simulink subsystem "Plant_PlantWithPressureBus"  (R2023a)
settings: Solver=VariableStepAuto  StartTime=0.0  StopTime=10.0  RelTol=1e-3
settings Model: Creator=giaco  LastModifiedBy=giaco

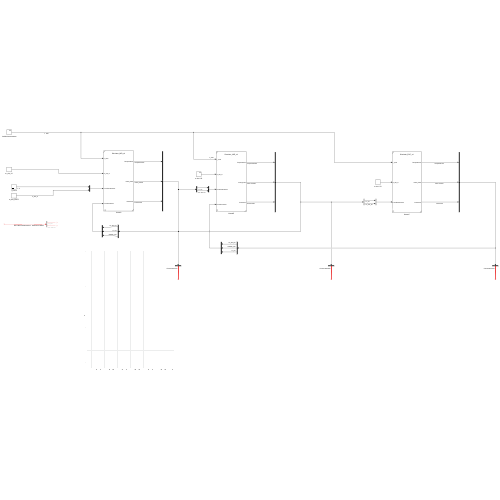
[thumbnail: Simulink's stored preview of the top-level diagram]
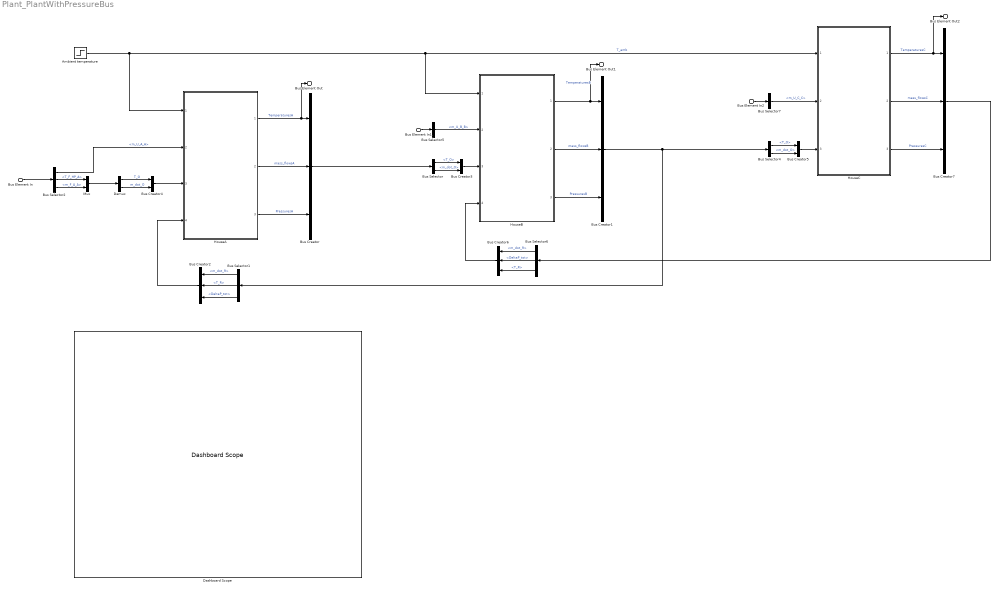
== system Plant_PlantWithPressureBus ==
  Bus Element In : Inport  PortName=InSim  Element=HouseA
  Bus Element In1 : Inport  PortName=InSim  Element=HouseB
  Bus Element In2 : Inport  PortName=InSim  Element=HouseC
  Ambient temperature : Step  Time=0  Before=300  After=300  SampleTime=0
  Bus Creator{,1..2,6..7} (5 alike) : BusCreator  Inputs=3
  Bus Creator3 : BusCreator  Inputs=2
  Bus Creator4 : BusCreator  Inputs=2
  Bus Creator5 : BusCreator  Inputs=2
  Bus Selector : BusSelector  OutputSignals=TemperaturesA.T_O,mass_flowsA.m_dot_O
  Bus Selector1 : BusSelector  OutputSignals=mass_flowsB.m_dot_R,TemperaturesB.T_R,PressuresB.DeltaP_tot
  Bus Selector2 : BusSelector  OutputSignals=m_U_A_A,T_F_HP_A,m_F_A_A
  Bus Selector4 : BusSelector  OutputSignals=TemperaturesB.T_O,mass_flowsB.m_dot_O
  Bus Selector5 : BusSelector  OutputSignals=m_U_B_B
  Bus Selector6 : BusSelector  OutputSignals=mass_flowsC.m_dot_R,PressuresC.DeltaP_tot,TemperaturesC.T_R
  Bus Selector7 : BusSelector  OutputSignals=m_U_C_C
  Dashboard Scope : DashboardScope
  Demux : Demux  Outputs=2
  HouseA : Subsystem  ReferencedSubsystem=Simulator_MID_v4  rho=971  c_p=4179  pi=3.14151  f_Darcy=0.025  L_F=40.5  D_F=0.4  h_F=1.5  D_S1=1  L_S1=0.4  h_S1=1.5  D_S2=0.4  L_S2=50  h_S2=1.5  D_S3=0.4  L_S3=5  h_S3=1.5  D_R=0.4  L_R=40  h_R=1.5  C_b=300  A_b=500  h_b=1.5  T_F_0=273  T_S1_0=273  T_S2_0=273  T_S3_0=273  T_b_0=273  T_R_0=273
  HouseB : Subsystem  ReferencedSubsystem=Simulator_MID_v4  rho=971  c_p=4179  pi=3.14151  f_Darcy=0.025  L_F=40.5  D_F=0.4  h_F=1.5  D_S1=1  L_S1=0.4  h_S1=1.5  D_S2=0.4  L_S2=50  h_S2=1.5  D_S3=0.4  L_S3=5  h_S3=1.5  D_R=0.4  L_R=40  h_R=1.5  C_b=300  A_b=500  h_b=1.5  T_F_0=273  T_S1_0=273  T_S2_0=273  T_S3_0=273  T_b_0=273  T_R_0=273
  HouseC : Subsystem  ReferencedSubsystem=Simulator_BYP_v4  rho=971  rho_air=971  c_p=4179  c_p_air=4179  pi=3.14151  f_Darcy=0.025  L_F=40.5  D_F=0.4  h_F=1.5  D_S1=0.4  L_S1=5  h_S1=1.5  D_S2=0.4  L_S2=5000  h_S2=300  D_S3=0.4  L_S3=5  h_S3=0.4  D_R=0.4  L_R=40  h_R=1.5  C_b=100  A_b=500  h_b=1.5  D_BYP=0.1  L_BYP=3  h_BYP=1.5  T_F_0=273  T_S1_0=273  T_S2_0=273  T_S3_0=273  T_b_0=273  T_R_0=273
  Mux : Mux  Inputs=2
  Bus Element Out : Outport  PortName=OutSim  Element=HouseA
  Bus Element Out1 : Outport  PortName=OutSim  Element=HouseB
  Bus Element Out2 : Outport  PortName=OutSim  Element=HouseC
  wires:
  Bus Selector1/1 -> Bus Creator2/1  "<m_dot_R>"
  HouseC/2 -> Bus Creator7/2  "mass_flowsC"
  Bus Selector6/1 -> Bus Creator6/1  "<m_dot_R>"
  Bus Selector1/3 -> Bus Creator2/3  "<DeltaP_tot>"
  Bus Creator4/1 -> HouseA/3
  Bus Selector6/2 -> Bus Creator6/2  "<DeltaP_tot>"
  Bus Selector6/3 -> Bus Creator6/3  "<T_R>"
  Bus Selector5/1 -> HouseB/2  "<m_U_B_B>"
  Bus Creator7/1 -> Bus Selector6/1
  Bus Creator6/1 -> HouseB/4
  Ambient temperature/1 -> HouseC/1, HouseB/1, HouseA/1  "T_amb"
  HouseC/1 -> Bus Creator7/1, Bus Element Out2/1  "TemperaturesC"
  Bus Creator3/1 -> HouseB/3
  Bus Selector4/2 -> Bus Creator5/2  "<m_dot_O>"
  Bus Creator2/1 -> HouseA/4
  Bus Selector4/1 -> Bus Creator5/1  "<T_O>"
  Bus Creator1/1 -> Bus Selector4/1, Bus Selector1/1
  HouseA/1 -> Bus Creator/1, Bus Element Out/1  "TemperaturesA"
  HouseB/2 -> Bus Creator1/2  "mass_flowsB"
  HouseA/2 -> Bus Creator/2  "mass_flowsA"
  Bus Selector/1 -> Bus Creator3/1  "<T_O>"
  Bus Selector/2 -> Bus Creator3/2  "<m_dot_O>"
  HouseB/1 -> Bus Creator1/1, Bus Element Out1/1  "TemperaturesB"
  Bus Creator/1 -> Bus Selector/1
  Bus Selector1/2 -> Bus Creator2/2  "<T_R>"
  HouseC/3 -> Bus Creator7/3  "PressuresC"
  Bus Creator5/1 -> HouseC/3
  HouseB/3 -> Bus Creator1/3  "PressuresB"
  Bus Selector7/1 -> HouseC/2  "<m_U_C_C>"
  HouseA/3 -> Bus Creator/3  "PressuresA"
  Bus Element In/1 -> Bus Selector2/1
  Bus Selector2/1 -> HouseA/2  "<m_U_A_A>"
  Bus Element In1/1 -> Bus Selector5/1
  Bus Element In2/1 -> Bus Selector7/1
  Mux/1 -> Demux/1
  Demux/1 -> Bus Creator4/1  "T_O"
  Demux/2 -> Bus Creator4/2  "m_dot_O"
  Bus Selector2/2 -> Mux/1  "<T_F_HP_A>"
  Bus Selector2/3 -> Mux/2  "<m_F_A_A>"
